simulink model "software1"  (Simulink 7.4)
settings: Solver=ode45  StartTime=0.0  StopTime=2  RelTol=1e-3
undefined symbols (not defined in the file or in its folder): des_figposition, get, One, sided
libraries: simeventssink1 x2, dspsrcs4 x1, dspsnks4 x1
settings Model: Creator=Chris  LastModifiedBy=Chris
settings SimEventsCC: propDiagAttribOutput=1  propDiagFcnCallOutput=1  propDiagStatOutput=0

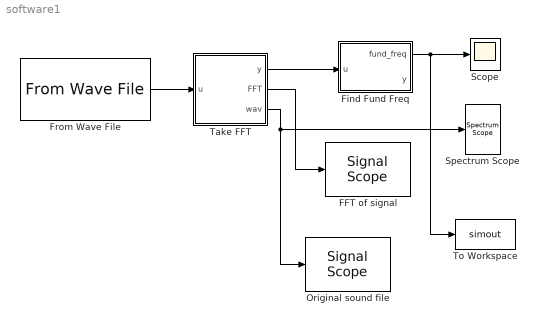
== system software1 ==
  FFT of signal : simeventssink1/Signal Scope  Priority=1  SystemSampleTime=-1  PlotType=Stair  InputType=Signal  NumInputs=1  AttributeNameY=Count  XInputOptionSignal=Event time  XInputOptionEntity=Event time  AttributeNameX=Count  EnableEntityOutport=on  XMin=0  XMax=2  XLimitExceededOption=Stretch axis limits  YLimitExceededOption=Stretch axis limits  AxisGrid=on  AxisLegend=off  LineDisables=""  LineColors=b  LineStyles=-  LineMarkers=.  OpenScopeAtSimStart=on  Title=FFT  YLabel=Amplitude  XLabel=Time  FigurePosition=des_figposition([5 60 25 25])  AxisZoom=off  DataStoreOption=Limited  DataPointsLimit=10000  StatNumberArrived=Off  ShowCountPlotted=off  ShowToolbar=on
      settings: YMin=0  YMax=14
  Find Fund Freq : Stateflow chart
  From Wave File : dspsrcs4/From Wave File  FileName=test1_222.wav  SamplesPerFrame=256  MinBufSize=256  dType=double  bLoop=off  timesToPlay=1  restartMode=immediately after last sample  firstSampleOutput=off  lastSampleOutput=off
  Original sound file : simeventssink1/Signal Scope  Priority=1  SystemSampleTime=-1  PlotType=Stair  InputType=Signal  NumInputs=1  AttributeNameY=Count  XInputOptionSignal=Event time  XInputOptionEntity=Event time  AttributeNameX=Count  EnableEntityOutport=on  XMin=0  XMax=2  XLimitExceededOption=Stretch axis limits  YLimitExceededOption=Stretch axis limits  AxisGrid=on  AxisLegend=off  LineDisables=""  LineColors=b  LineStyles=-  LineMarkers=.  OpenScopeAtSimStart=on  Title=Original .wav sound file  YLabel=Amplitude  XLabel=Time  FigurePosition=des_figposition([5 60 25 25])  AxisZoom=off  DataStoreOption=Limited  DataPointsLimit=10000  StatNumberArrived=Off  ShowCountPlotted=off  ShowToolbar=on
      settings: YMin=-2  YMax=2
  Scope : Scope
  Spectrum Scope : dspsnks4/Spectrum Scope  DialogController=dspdialog.SpectrumScope  DialogControllerArgs=DataTag2  SystemSampleTime=-1  ScopeProperties=on  Domain=Frequency  HorizSpan=1  UseBuffer=on  BufferSize=128  Overlap=64  inpFftLenInherit=off  FFTlength=128  numAvg=2  DisplayProperties=off  AxisGrid=on  Memory=off  FrameNumber=on  AxisLegend=off  AxisZoom=off  OpenScopeAtSimStart=on  OpenScopeImmediately=off  FigPos=get(0,'defaultfigureposition')  AxisProperties=off  XUnits=Hertz  XRange=One-sided ([0...Fs/2])  XDisplay=0  InheritXIncr=on  XIncr=1.0  XLabel=Samples  XLimit=Auto  YUnits=dBW  XMax=1  XMin=0  YLabel=Magnitude-squared, dB  LineProperties=off  LineStyles=-  wintypeSpecScope=Hann  RsSpecScope=50  betaSpecScope=5  winsampSpecScope=Periodic  XAxisParamsVer=6.9
      settings: YMin=-10  YMax=10
  Take FFT : Stateflow chart
  To Workspace : ToWorkspace  VariableName=simout  SampleTime=-1  SaveFormat=Structure
  wires:
  From Wave File/1 -> Take FFT/1(u)
  Take FFT/1(y) -> Find Fund Freq/1(u)
  Find Fund Freq/1(fund_freq) -> Scope/1, To Workspace/1
  Take FFT/2(FFT) -> FFT of signal/1
  Take FFT/3(wav) -> Original sound file/1, Spectrum Scope/1

== matlab function Find Fund Freq ==
  data: u input double; fund_freq output double size=1,1 [0..99999999]; y output double
function [fund_freq, y]= fcn(u)
%#em2
%Chris Jagielski
%Find Fundamental Frequency!

y = u; %retain spectrum

value = max(u); %peak in frequency domain
a = find(u==value,1,'first')-1; %finds only 1 value that matches
fund_freq = a(1,1);

== matlab function Take FFT ==
  data: u input double; y output double; FFT output double; wav output double
function [y,FFT,wav]  = fcn(u)
%#em1
%Chris Jagielski

L = length(u);
wav = u(L,1); %ORIGINAL sound

y = abs(fft(u)); %obtain real values only of FFT of sound
l = length(y);
FFT = y(l,1); %the frequency domain of it?

% l = length(u);
% wav = u(l,1); %the original input .wav file
